simulink model "test"  (Simulink 7.5)
settings: Solver=ode15s  StartTime=0.0  StopTime=10  RelTol=1e-3
libraries: powerlib x3, simulink x1
settings Model: Creator=lm  LastModifiedBy=lm

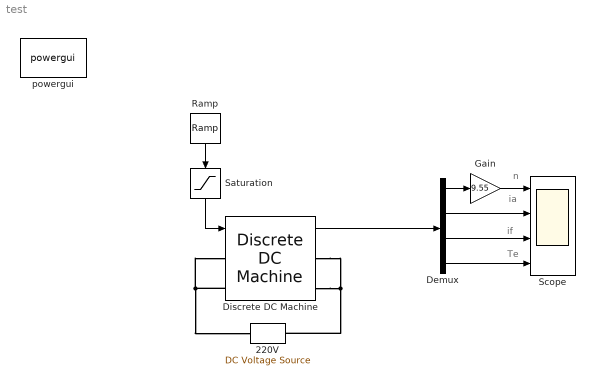
== system test ==
  note: n
  note: ia
  note: if
  note: Te
  220V : powerlib/Electrical Sources/DC Voltage Source  DialogController=POWERSYS.PowerSysDialog  SystemSampleTime=-1  Amplitude=220  Measurements=None
  Demux : Demux
  Discrete DC Machine : powerlib/Machines/Discrete DC Machine  DialogController=POWERSYS.PowerSysDialog  SystemSampleTime=-1  PresetModel=No  MechanicalLoad=Torque TL  FieldType=Wound  ShowDetailedParameters=on  RLa="[ 0.21  0.000021]"  RLf=[ 146.7 0]  Laf=0.84  MachineConstant=Torque constant (N.m/A)  Ke=1.8  Kt=1.8  J=0.57  Bm=0  Tf=0  w0=0  Ifinit=1  TsPowergui=0  TsBlock=-1
      settings: AttributesFormatString=\n
  Gain : Gain  Gain=9.55  ParameterDataType=fixdt(1, 16)  ParameterScaling=2^0  OutDataType=fixdt(1, 16)  OutScaling=2^0
  Ramp : simulink/Sources/Ramp  SystemSampleTime=-1  slope=100000  start=2.5  X0=0
  Saturation : Saturate  UpperLimit=171  LowerLimit=0  LinearizeAsGain=off  OutDataType=fixdt(1, 16)  OutScaling=2^0
  Scope : Scope  NumInputPorts=4
      settings: YMin=1680.6~-0.0034~1.42468~-0.00425  YMax=1682~-0.00285~1.57464~-0.0036
  powergui : powerlib/powergui  Priority=1  SystemSampleTime=-1  SimulationMode=Continuous  SampleTime=50e-6  frequency=60  SPID=off  DisableSnubberDevices=off  DisableRonSwitches=off  DisableVfSwitches=off  SwTol=0  Interpol=off  frequencyindice=0  echomessages=off  HookPort=off  DisplayEquations=off  FunctionMessages=off  EnableUseOfTLC=off  x0status=blocks  RestoreLinks=warning  ResistiveCurrentMeasurement=off  Ylog=off  Xlog=on  ShowGrid=off  save=off  variable=ZData  ZoomFFT=off  StartTime=0.0  cycles=1  DisplayStyle=1  FreqAxis=off  MaxFrequency=1000  frequencyindicesteady=1  display=off  methode=off
  wires:
  Ramp/1 -> Saturation/1
  Demux/2 -> Scope/2
  Demux/3 -> Scope/3
  Demux/4 -> Scope/4
  Demux/1 -> Gain/1
  Gain/1 -> Scope/1
  Discrete DC Machine/1 -> Demux/1
  Saturation/1 -> Discrete DC Machine/1
  connections:
  Discrete DC Machine/LConn2 -- 220V/RConn1 -- Discrete DC Machine/LConn1
  Discrete DC Machine/RConn2 -- 220V/LConn1 -- Discrete DC Machine/RConn1
